simulink model "test"  (R2022b)
settings: Solver=VariableStepAuto  StartTime=0.0  StopTime=20  RelTol=1e-3
settings Model: Creator=micky  LastModifiedBy=micky

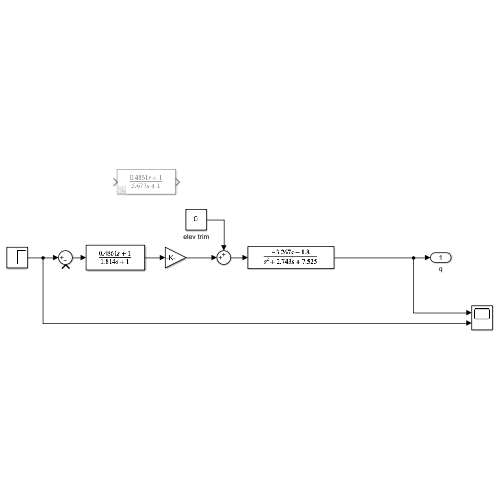
[thumbnail: Simulink's stored preview of the top-level diagram]
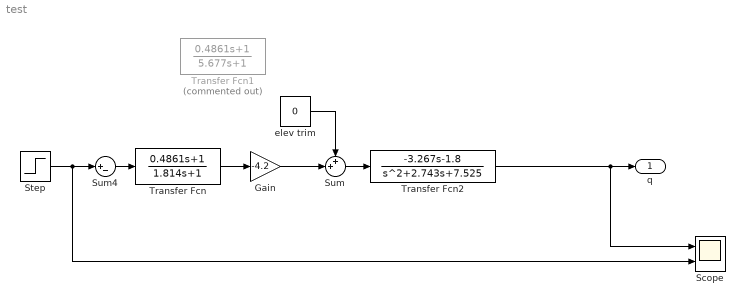
== system test ==
  Gain : Gain  Gain=-4.2
  Scope : Scope  NumInputPorts=2
  Step : Step  Time=5  SampleTime=0
  Sum : Sum  Inputs=++|
  Sum4 : Sum  Inputs=|+-
  Transfer Fcn : TransferFcn  Numerator=[0.4861 1]  Denominator=[1.814 1]
  Transfer Fcn1 : TransferFcn  Commented=on  Numerator=[0.4861 1]  Denominator=[5.677 1]
  Transfer Fcn2 : TransferFcn  Numerator=[-3.267 -1.8]  Denominator=[1 2.743 7.525]
  elev trim : Constant  Value=0
  q : Outport
  wires:
  Transfer Fcn2/1 -> Scope/1, q/1
  Step/1 -> Scope/2, Sum4/1
  Sum4/1 -> Transfer Fcn/1
  Gain/1 -> Sum/2
  Sum/1 -> Transfer Fcn2/1
  elev trim/1 -> Sum/1
  Transfer Fcn/1 -> Gain/1
